simulink model "PQ_GRUPOB_trajetorias_v_i_motor"  (R2018a)
settings: Solver=VariableStepAuto  StartTime=0.0  StopTime=1  RelTol=1e-3
libraries: powerlib x15, powerlib_meascontrol x1
settings Model: Creator=Rafael Pavan  LastModifiedBy=Rafael Pavan

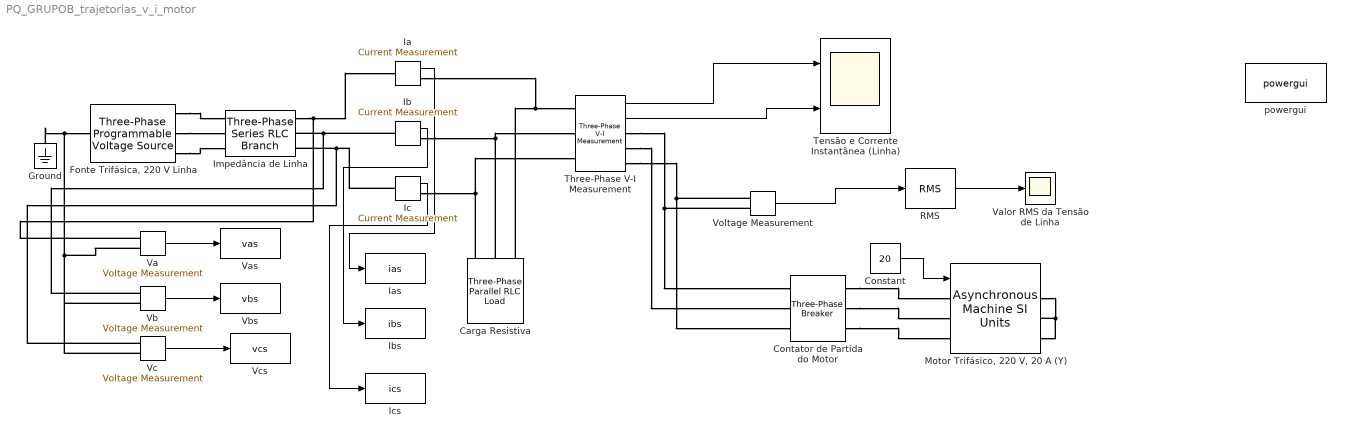
== system PQ_GRUPOB_trajetorias_v_i_motor ==
  Carga Resistiva : powerlib/Elements/Three-Phase Parallel RLC Load  LConnTagsString=A|B|C  Configuration=Y (grounded)  NominalVoltage=220  Vabc=[1e3 1e3 1e3]  Vabcp=[1e3 1e3 1e3]  NominalFrequency=60  UnbalancedPower=off  ActivePower=500  InductivePower=0  CapacitivePower=0  Pabc=[10e3 9e3 11e3]  QLabc=[100 90 110]  QCabc=[100 90 110]  Pabcp=[10e3 9e3 11e3]  QLabcp=[100 90 110]  QCabcp=[100 90 110]  Measurements=None  LoadType=constant Z
  Constant : Constant  Value=20
  Contator de Partida do Motor : powerlib/Elements/Three-Phase Breaker  InitialState=open  SwitchA=on  SwitchB=on  SwitchC=on  SwitchTimes=[0.2 15]  External=off  BreakerResistance=0.01  SnubberResistance=1e6  SnubberCapacitance=inf  Measurements=None
  "Fonte Trifásica, 220 V Linha " : powerlib/Electrical Sources/Three-Phase Programmable Voltage Source  PositiveSequence=[220 0 60]  VariationEntity=None  VariationType=Table of time-amplitude pairs  VariationTypeAlt=Step  VariationStep=0.5  VariationRate=10  VariationMagnitude=0.3  VariationFrequency=2  VariationTiming=[1 2]  VariationPhaseA=off  Amplitudes=[1 0.8 1.2 1.0]  TimeValues=[0 0.1 0.15 0.2]  HarmonicGeneration=off  HarmonicA=[3 0.2 -25 0]  HarmonicB=[2 0.15 35 2]  Timing="[0.05  3]"  BusType=PV  Pref=1000000000  Qref=0  Qmin=-inf  Qmax=inf
  Ground : powerlib/Elements/Ground  LConnTagsString=a
  Ia : powerlib/Measurements/Current Measurement  PhasorSimulation=off  OutputType=Complex  PSBequivalent=0
  Ias : ToWorkspace  VariableName=ias  SampleTime=-1
  Ib : powerlib/Measurements/Current Measurement  PhasorSimulation=off  OutputType=Complex  PSBequivalent=0
  Ibs : ToWorkspace  VariableName=ibs  SampleTime=-1
  Ic : powerlib/Measurements/Current Measurement  PhasorSimulation=off  OutputType=Complex  PSBequivalent=0
  Ics : ToWorkspace  VariableName=ics  SampleTime=-1
  "Impedância de Linha " : powerlib/Elements/Three-Phase Series RLC Branch  LConnTagsString=A|B|C  RConnTagsString=A|B|C  BranchType=RL  Resistance=0.0001  Inductance=1e-3  Capacitance=1e-2  Measurements=None
  "Motor Trifásico, 220 V, 20 A (Y) " : powerlib/Machines/Asynchronous Machine SI Units  RotorType=Wound  PresetModel=No  MechanicalLoad=Torque Tm  ShowDetailedParameters=on  ReferenceFrame=Rotor  Units=SI  MeasurementBus=off  NominalParameters=[7612 220 60]  Stator=[0.5968 0.0003495]  Rotor=[0.6258 0.005473]  Cage1=[0.4155 0.002066]  Cage2=[0.4168 0.0003495]  Lm=0.0354  Mechanical=[0.05 0.005879 4]  PolePairs=2  InitialConditions=[0 0 0 0 0 0 0 0]  SimulateSaturation=off  Saturation=[14.03593122, 27.81365428, 53.79336849, 72.68890987, 97.98006896, 148.6815601, 215.7428561, 302.9841135, 428.7778367 ; 230, 322, 414, 460, 506, 552, 598, 644, 690]  LoadFlowParameters=1492000  TsPowergui=0  TsBlock=-1  IterativeModel=Trapezoidal non iterative  IterativeDiscreteModel=Trapezoidal non iterative  Pmec=5709
  RMS : powerlib_meascontrol/Measurements/RMS  TrueRMS=on  Freq=60  RMSInit=220  Ts=0
  Tensão e Corrente Instantânea (Linha) : Scope  NumInputPorts=2
  Three-Phase V-I Measurement : powerlib/Measurements/Three-Phase V-I Measurement  VoltageMeasurement=phase-to-ground  SetLabelV=off  LabelV=Vabc  Vpu=off  VpuLL=off  CurrentMeasurement=yes  SetLabelI=off  LabelI=Iabc  Ipu=off  Pbase=100e6  Vbase=220  OutputType=Complex  PhasorSimulation=off  PSBequivalent=0
  Va : powerlib/Measurements/Voltage Measurement  PhasorSimulation=off  OutputType=Complex  PSBequivalent=0
  Valor RMS da Tensão de Linha : Scope
  Vas : ToWorkspace  VariableName=vas  SampleTime=-1
  Vb : powerlib/Measurements/Voltage Measurement  PhasorSimulation=off  OutputType=Complex  PSBequivalent=0
  Vbs : ToWorkspace  VariableName=vbs  SampleTime=-1
  Vc : powerlib/Measurements/Voltage Measurement  PhasorSimulation=off  OutputType=Complex  PSBequivalent=0
  Vcs : ToWorkspace  VariableName=vcs  SampleTime=-1
  Voltage Measurement : powerlib/Measurements/Voltage Measurement  PhasorSimulation=off  OutputType=Complex  PSBequivalent=0
  powergui : powerlib/powergui  Priority=1  SimulationMode=Continuous  SampleTime=50e-6  frequency=60  Iterations=50  frequencyindice=60  Pbase=100e6  ErrMax=1e-4  UnitsV=kV  UnitsW=MW  buscounter=0  FunctionMessages=on  echomessages=off  EnableUseOfTLC=off  CurrentSourceSwitches=off  DisableSnubberDevices=off  DisableRonSwitches=off  DisableVfSwitches=off  DisplayEquations=off  SolverType=Tustin/Backward Euler (TBE)  Interpol=off  ExternalGateDelay=off  methode=off  Ts=100  x0status=blocks  SPID=on  SwTol=0  HookPort=off  RestoreLinks=warning  ResistiveCurrentMeasurement=off  Frange=[0:2:500]  Ylog=off  Xlog=on  ShowGrid=off  save=off  variable=ZData  structure=0  ZoomFFT=off  StartTime=0.0  cycles=1  DisplayStyle=1  fundamental=60  FreqAxis=off  MaxFrequency=1000  frequencyindicesteady=1  RmsSteady=1  display=off
  wires:
  Constant/1 -> "Motor Trifásico, 220 V, 20 A (Y) "/1
  Three-Phase V-I Measurement/1 -> Tensão e Corrente Instantânea (Linha)/1
  Voltage Measurement/1 -> RMS/1
  RMS/1 -> Valor RMS da Tensão de Linha/1
  Three-Phase V-I Measurement/2 -> Tensão e Corrente Instantânea (Linha)/2
  Ia/1 -> Ias/1
  Ib/1 -> Ibs/1
  Ic/1 -> Ics/1
  Va/1 -> Vas/1
  Vb/1 -> Vbs/1
  Vc/1 -> Vcs/1
  connections:
  "Motor Trifásico, 220 V, 20 A (Y) "/RConn1 -- "Motor Trifásico, 220 V, 20 A (Y) "/RConn3 -- "Motor Trifásico, 220 V, 20 A (Y) "/RConn2
  Contator de Partida do Motor/RConn1 -- "Motor Trifásico, 220 V, 20 A (Y) "/LConn1
  Contator de Partida do Motor/RConn2 -- "Motor Trifásico, 220 V, 20 A (Y) "/LConn2
  Contator de Partida do Motor/RConn3 -- "Motor Trifásico, 220 V, 20 A (Y) "/LConn3
  "Fonte Trifásica, 220 V Linha "/RConn1 -- "Impedância de Linha "/LConn1
  "Fonte Trifásica, 220 V Linha "/RConn2 -- "Impedância de Linha "/LConn2
  "Fonte Trifásica, 220 V Linha "/RConn3 -- "Impedância de Linha "/LConn3
  Carga Resistiva/LConn2 -- Ib/RConn1 -- Three-Phase V-I Measurement/LConn2
  Carga Resistiva/LConn3 -- Ia/RConn1 -- Three-Phase V-I Measurement/LConn1
  Carga Resistiva/LConn1 -- Ic/RConn1 -- Three-Phase V-I Measurement/LConn3
  Three-Phase V-I Measurement/RConn3 -- Voltage Measurement/LConn1 -- Contator de Partida do Motor/LConn3
  Three-Phase V-I Measurement/RConn2 -- Contator de Partida do Motor/LConn2
  Three-Phase V-I Measurement/RConn1 -- Voltage Measurement/LConn2 -- Contator de Partida do Motor/LConn1
  Ib/LConn1 -- Vb/LConn1 -- "Impedância de Linha "/RConn2
  "Impedância de Linha "/RConn1 -- Va/LConn1 -- Ia/LConn1
  Ic/LConn1 -- Vc/LConn1 -- "Impedância de Linha "/RConn3
  Ground/LConn1 -- Vb/LConn2 -- Vc/LConn2 -- Va/LConn2 -- "Fonte Trifásica, 220 V Linha "/LConn1
